simulink model "LKF"  (R2012b)
settings: Solver=ode3  StartTime=0.0  StopTime=SimulStop  FixedStep=0.05  RelTol=1e-3
undefined symbols (not defined in the file or in its folder): A, A1, C, P_init, SimulStop, T1, V1, W1, xhat_init
libraries: dspmtrx3 x4, commnoisgen2 x1, dspinverses x1
settings Model: Creator=DonghanLee  LastModifiedBy=DonghanLee

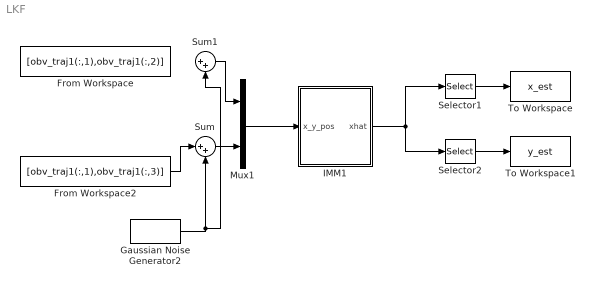
== system LKF ==
  From Workspace : FromWorkspace  VariableName=[obv_traj1(:,1),obv_traj1(:,2)]  SampleTime=0
  From Workspace2 : FromWorkspace  VariableName=[obv_traj1(:,1),obv_traj1(:,3)]  SampleTime=0
  Gaussian Noise Generator2 : commnoisgen2/Gaussian Noise Generator  m=0  d=noise  s=0  Ts=0.05  frameBased=off  sampPerFrame=1  orient=off  outDataType=double
  IMM1 : Subsystem
  Mux1 : Mux  Inputs=2
  Selector1 : Selector  InputPortWidth=4  IndexOptions=Index vector (dialog)  Indices=[1 2]  OutputSizes=1
  Selector2 : Selector  InputPortWidth=4  IndexOptions=Index vector (dialog)  Indices=[3 4]  OutputSizes=1
  Sum : Sum  Inputs=|++
  Sum1 : Sum  Inputs=|++
  To Workspace : ToWorkspace  VariableName=x_est  SampleTime=-1
  To Workspace1 : ToWorkspace  VariableName=y_est  SampleTime=-1
  wires:
  Mux1/1 -> IMM1/1(x_y_pos)
  Gaussian Noise Generator2/1 -> Sum1/2, Sum/2
  From Workspace2/1 -> Sum/1
  Sum/1 -> Mux1/2
  Sum1/1 -> Mux1/1
  IMM1/1(xhat) -> Selector2/1, Selector1/1
  Selector1/1 -> To Workspace/1
  Selector2/1 -> To Workspace1/1

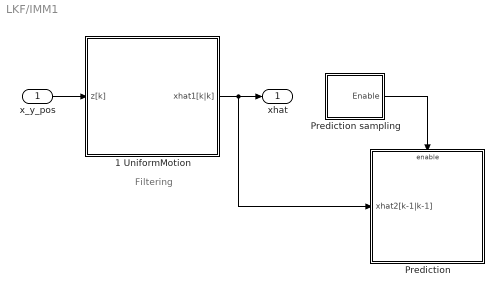
== system LKF/IMM1 ==
  note: Filtering
  x_y_pos : Inport
  "1 UniformMotion " : Subsystem
  Prediction : Subsystem
  Prediction sampling : Subsystem
  xhat : Outport
  wires:
  x_y_pos/1 -> "1 UniformMotion "/1(z[k])
  "1 UniformMotion "/1(xhat1[k|k]) -> Prediction/1(xhat2[k-1|k-1]), xhat/1
  Prediction sampling/1(Enable) -> Prediction/Enable

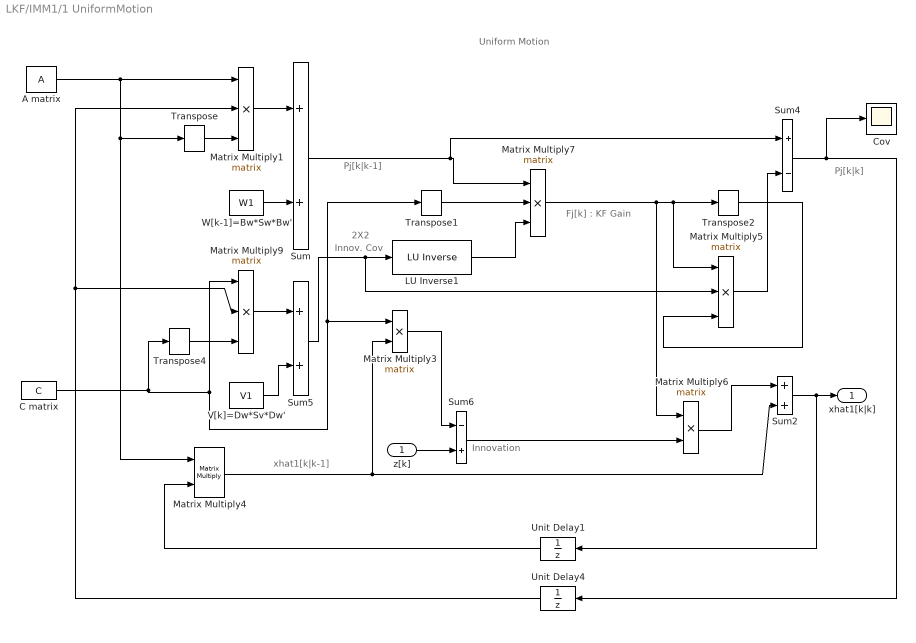
== system LKF/IMM1/1 UniformMotion  ==
  note: 2X2
  note: Pj[k|k]
  note: Innovation
  note: Innov. Cov
  note: Pj[k|k-1]
  note: xhat1[k|k-1]
  note: Uniform Motion
  note: Fj[k] : KF Gain
  z[k] : Inport
  " LU Inverse1" : dspinverses/ LU Inverse
  A matrix : Constant  Value=A
  C matrix : Constant  Value=C
  Cov : Scope
      settings: SaveName=ScopeData3
  Matrix Multiply{1,5,7,9} (4 alike) : Product  Inputs=3  Multiplication=Matrix(*)
  Matrix Multiply3 : Product  Multiplication=Matrix(*)
  Matrix Multiply4 : Product  Multiplication=Matrix(*)
  Matrix Multiply6 : Product  Multiplication=Matrix(*)
  Sum : Sum  SaturateOnIntegerOverflow=on
  Sum2 : Sum  SaturateOnIntegerOverflow=on
  Sum4 : Sum  Inputs=+-  SaturateOnIntegerOverflow=on
  Sum5 : Sum  SaturateOnIntegerOverflow=on
  Sum6 : Sum  Inputs=-+  SaturateOnIntegerOverflow=on
  Transpose{,1..2,4} (4 alike) : dspmtrx3/Transpose  Hermitian=off  overflowFlag=off
  Unit Delay1 : UnitDelay  InitialCondition=xhat_init  SampleTime=-1
  Unit Delay4 : UnitDelay  InitialCondition=P_init  SampleTime=-1
  V[k]=Dw*Sv*Dw' : Constant  Value=V1
  "W[k-1]=Bw*Sw*Bw' " : Constant  Value=W1
  xhat1[k|k] : Outport
  wires:
  Transpose/1 -> Matrix Multiply1/3
  A matrix/1 -> Matrix Multiply1/1, Matrix Multiply4/1, Transpose/1
  Matrix Multiply1/1 -> Sum/1
  Matrix Multiply3/1 -> Sum6/1
  C matrix/1 -> Transpose4/1, Matrix Multiply9/1, Transpose1/1, Matrix Multiply3/1
  Matrix Multiply4/1 -> Matrix Multiply3/2, Sum2/2
  Matrix Multiply7/1 -> Matrix Multiply6/1, Matrix Multiply5/1, Transpose2/1
  Transpose2/1 -> Matrix Multiply5/3
  Matrix Multiply6/1 -> Sum2/1
  Sum2/1 -> Unit Delay1/1, xhat1[k|k]/1
  "W[k-1]=Bw*Sw*Bw' "/1 -> Sum/2
  Sum4/1 -> Cov/1, Unit Delay4/1
  Sum5/1 -> Matrix Multiply5/2, " LU Inverse1"/1
  " LU Inverse1"/1 -> Matrix Multiply7/3
  Unit Delay4/1 -> Matrix Multiply1/2, Matrix Multiply9/2
  Transpose4/1 -> Matrix Multiply9/3
  Matrix Multiply9/1 -> Sum5/1
  V[k]=Dw*Sv*Dw'/1 -> Sum5/2
  Transpose1/1 -> Matrix Multiply7/2
  z[k]/1 -> Sum6/2
  Sum6/1 -> Matrix Multiply6/2
  Matrix Multiply5/1 -> Sum4/2
  Sum/1 -> Sum4/1, Matrix Multiply7/1
  Unit Delay1/1 -> Matrix Multiply4/2

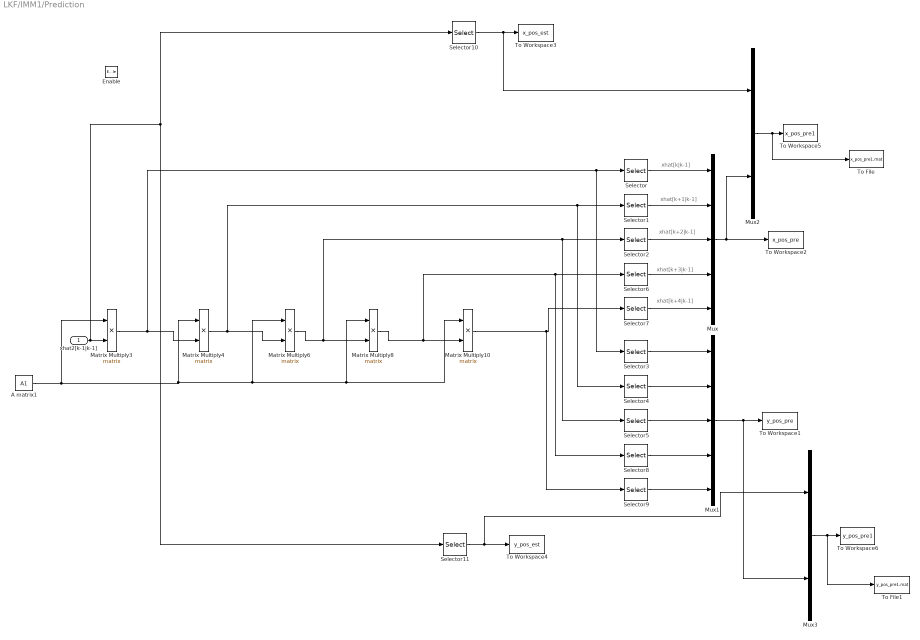
== system LKF/IMM1/Prediction ==
  note: xhat[k+3|k-1]
  note: xhat[k+2|k-1]
  note: xhat[k|k-1]
  note: xhat[k+1|k-1]
  note: xhat[k+4|k-1]
  xhat2[k-1|k-1] : Inport
  Enable : EnablePort
  A matrix1 : Constant  Value=A1
  Matrix Multiply{3..4,6,8,10} (5 alike) : Product  Multiplication=Matrix(*)
  Mux : Mux  Inputs=5
  Mux1 : Mux  Inputs=5
  Mux2 : Mux  Inputs=2
  Mux3 : Mux  Inputs=2
  Selector{,1..2,6..7,10} (6 alike) : Selector  InputPortWidth=4  IndexOptions=Index vector (dialog)  Indices=[1]  OutputSizes=1
  Selector{3..5,8..9,11} (6 alike) : Selector  InputPortWidth=4  IndexOptions=Index vector (dialog)  Indices=[3]  OutputSizes=1
  To File : ToFile  Filename=x_pos_pre1.mat  MatrixName=x_pos_pre1
  To File1 : ToFile  Filename=y_pos_pre1.mat  MatrixName=y_pos_pre1
  To Workspace1 : ToWorkspace  VariableName=y_pos_pre  SampleTime=-1
  To Workspace2 : ToWorkspace  VariableName=x_pos_pre  SampleTime=-1
  To Workspace3 : ToWorkspace  VariableName=x_pos_est  SampleTime=-1
  To Workspace4 : ToWorkspace  VariableName=y_pos_est  SampleTime=-1
  To Workspace5 : ToWorkspace  VariableName=x_pos_pre1  SampleTime=-1
  To Workspace6 : ToWorkspace  VariableName=y_pos_pre1  SampleTime=-1
  wires:
  Matrix Multiply3/1 -> Selector3/1, Selector/1, Matrix Multiply4/2
  Matrix Multiply4/1 -> Selector4/1, Selector1/1, Matrix Multiply6/2
  Matrix Multiply6/1 -> Selector5/1, Selector2/1, Matrix Multiply8/2
  Mux/1 -> Mux2/2, To Workspace2/1
  Mux1/1 -> Mux3/2, To Workspace1/1
  Matrix Multiply8/1 -> Selector8/1, Selector6/1, Matrix Multiply10/2
  Selector6/1 -> Mux/4
  Selector2/1 -> Mux/3
  Selector7/1 -> Mux/5
  Selector/1 -> Mux/1
  Selector1/1 -> Mux/2
  Selector3/1 -> Mux1/1
  Selector4/1 -> Mux1/2
  Selector5/1 -> Mux1/3
  Selector8/1 -> Mux1/4
  Selector9/1 -> Mux1/5
  A matrix1/1 -> Matrix Multiply3/1, Matrix Multiply6/1, Matrix Multiply8/1, Matrix Multiply10/1, Matrix Multiply4/1
  Matrix Multiply10/1 -> Selector9/1, Selector7/1
  xhat2[k-1|k-1]/1 -> Matrix Multiply3/2, Selector11/1, Selector10/1
  Selector10/1 -> Mux2/1, To Workspace3/1
  Selector11/1 -> Mux3/1, To Workspace4/1
  Mux2/1 -> To File/1, To Workspace5/1
  Mux3/1 -> To File1/1, To Workspace6/1

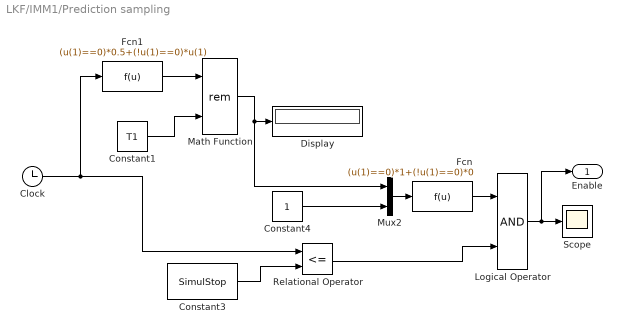
== system LKF/IMM1/Prediction sampling ==
  Clock : Clock
  Constant1 : Constant  Value=T1
  Constant3 : Constant  Value=SimulStop
  Constant4 : Constant
  Display : Display
  Fcn : Fcn  Expr=(u(1)==0)*1+(!u(1)==0)*0
  Fcn1 : Fcn  Expr=(u(1)==0)*0.5+(!u(1)==0)*u(1)
  Logical Operator : Logic  AllPortsSameDT=off  OutDataTypeStr=boolean
  Math Function : Math  Operator=rem  SaturateOnIntegerOverflow=on
  Mux2 : Mux  Inputs=2
  Relational Operator : RelationalOperator  Operator=<=  OutDataTypeStr=boolean
  Scope : Scope
      settings: SaveName=ScopeData2
  Enable : Outport
  wires:
  Clock/1 -> Fcn1/1, Relational Operator/1
  Constant1/1 -> Math Function/2
  Math Function/1 -> Mux2/1, Display/1
  Logical Operator/1 -> Enable/1, Scope/1
  Fcn/1 -> Logical Operator/1
  Relational Operator/1 -> Logical Operator/2
  Constant3/1 -> Relational Operator/2
  Constant4/1 -> Mux2/2
  Mux2/1 -> Fcn/1
  Fcn1/1 -> Math Function/1
